simulink model "assignment_2_simulink_q710"  (R2023a)
settings: Solver=VariableStepAuto  StartTime=0.0  StopTime=0.5  MaxStep=1e-4  RelTol=1e-3
values from neighbouring files (symbols this model uses):
  J = 1e-3    (= 0.001)    [assignment_2_script_q6.m]    (also in assignment_2_script_q710.m)
  k = 0.35    [assignment_2_script_q6.m]    (also in assignment_2_script_q710.m)
  k_i = alpha_c^2 * L    (= 15791.3670417)    [assignment_2_script_q6.m]    (also in assignment_2_script_q710.m = 11053.9569292)
  k_is = alpha_s^2 * J    (= 63.165468167)    [assignment_2_script_q6.m]    (also in assignment_2_script_q710.m = 0)
  k_p = 2 * alpha_c* L - R    (= 12.0663706144)    [assignment_2_script_q6.m]    (also in assignment_2_script_q710.m = 8.04645943005)
  k_ps = 2 * alpha_s * J    (= 0.502654824574)    [assignment_2_script_q6.m]    (also in assignment_2_script_q710.m = 0.251327412287)
  k_t = alpha_c * L    (= 6.28318530718)    [assignment_2_script_q6.m]    (also in assignment_2_script_q710.m = 4.39822971503)
  k_ts = alpha_s * J    (= 0.251327412287)    [assignment_2_script_q6.m]    (also in assignment_2_script_q710.m)
  L = 2.5e-3    (= 0.0025)    [assignment_2_script_q6.m]    (also in assignment_2_script_q710.m = 0.00175)
  R = 0.5    [assignment_2_script_q6.m]    (also in assignment_2_script_q710.m = 0.75)
  tau_max = 2*tau_N    (= 14)    [assignment_2_script_q6.m]    (also in assignment_2_script_q710.m)
  tau_min = -2*tau_N    (= -14)    [assignment_2_script_q6.m]    (also in assignment_2_script_q710.m)
  u_max = 140    [assignment_2_script_q6.m]    (also in assignment_2_script_q710.m)
  u_min = -140    [assignment_2_script_q6.m]    (also in assignment_2_script_q710.m)
settings Model: Creator=chowd  LastModifiedBy=chowd
settings DataIOCC: ReturnWorkspaceOutputs=off

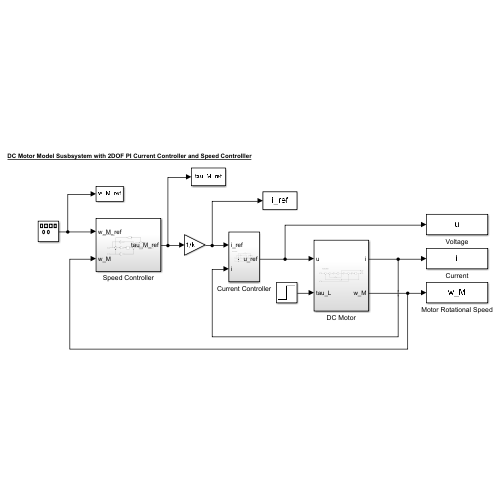
[thumbnail: Simulink's stored preview of the top-level diagram]
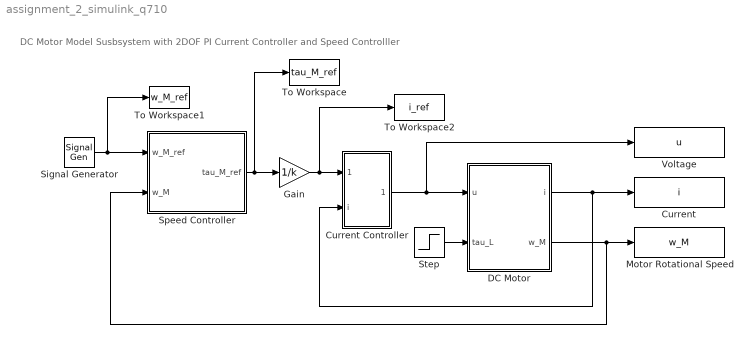
== system assignment_2_simulink_q710 ==
  note: DC Motor Model Susbsystem with 2DOF PI Current Controller and Speed Controlller
  Current : ToWorkspace  VariableName=i  SaveFormat=Timeseries  SampleTime=-1
  Current Controller : Subsystem
  DC Motor : Subsystem
  Gain : Gain  Gain=1/k
  Motor Rotational Speed : ToWorkspace  VariableName=w_M  SaveFormat=Timeseries  SampleTime=-1
  Signal Generator : SignalGenerator  WaveForm=square  Amplitude=160  Frequency=4
  Speed Controller : Subsystem
  Step : Step  Time=0.3  After=7  SampleTime=1
  To Workspace : ToWorkspace  VariableName=tau_M_ref  SaveFormat=Timeseries  SampleTime=-1
  To Workspace1 : ToWorkspace  VariableName=w_M_ref  SaveFormat=Timeseries  SampleTime=-1
  To Workspace2 : ToWorkspace  VariableName=i_ref  SaveFormat=Timeseries  SampleTime=-1
  Voltage : ToWorkspace  VariableName=u  SaveFormat=Timeseries  SampleTime=-1
  wires:
  Step/1 -> DC Motor/2(tau_L)
  Gain/1 -> To Workspace2/1, Current Controller/1(i_ref)
  DC Motor/1(i) -> Current/1, Current Controller/2(i)
  Current Controller/1(u_ref) -> Voltage/1, DC Motor/1(u)
  DC Motor/2(w_M) -> Speed Controller/2(w_M), Motor Rotational Speed/1
  Speed Controller/1(tau_M_ref) -> To Workspace/1, Gain/1
  Signal Generator/1 -> To Workspace1/1, Speed Controller/1(w_M_ref)

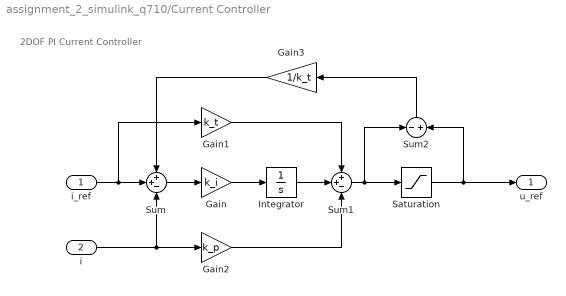
== system assignment_2_simulink_q710/Current Controller ==
  note: 2DOF PI Current Controller
  i_ref : Inport
  i : Inport  Port=2
  Gain : Gain  Gain=k_i
  Gain1 : Gain  Gain=k_t
  Gain2 : Gain  Gain=k_p
  Gain3 : Gain  Gain=1/k_t
  Integrator : Integrator
  Saturation : Saturate  UpperLimit=u_max  LowerLimit=u_min
  Sum : Sum  Inputs=++-
  Sum1 : Sum  Inputs=++-
  Sum2 : Sum  Inputs=-|+
  u_ref : Outport
  wires:
  i_ref/1 -> Sum/2, Gain1/1
  Saturation/1 -> u_ref/1, Sum2/2
  Gain3/1 -> Sum/1
  Integrator/1 -> Sum1/2
  Gain/1 -> Integrator/1
  Sum1/1 -> Sum2/1, Saturation/1
  Gain1/1 -> Sum1/1
  i/1 -> Sum/3, Gain2/1
  Sum/1 -> Gain/1
  Gain2/1 -> Sum1/3
  Sum2/1 -> Gain3/1

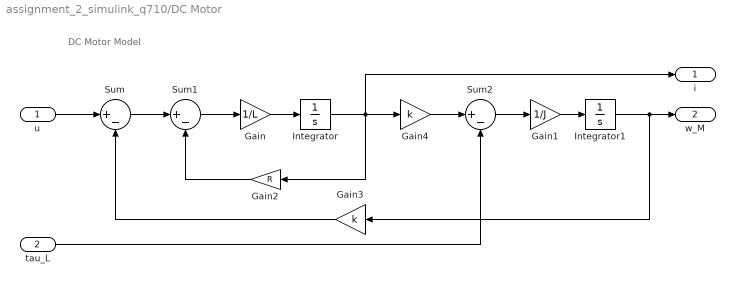
== system assignment_2_simulink_q710/DC Motor ==
  note: DC Motor Model
  u : Inport
  tau_L : Inport  Port=2
  Gain : Gain  Gain=1/L
  Gain1 : Gain  Gain=1/J
  Gain2 : Gain  Gain=R
  Gain3 : Gain  Gain=k
  Gain4 : Gain  Gain=k
  Integrator : Integrator
  Integrator1 : Integrator
  Sum : Sum  Inputs=|+-
  Sum1 : Sum  Inputs=|+-
  Sum2 : Sum  Inputs=|+-
  i : Outport
  w_M : Outport  Port=2
  wires:
  Gain/1 -> Integrator/1
  Sum2/1 -> Gain1/1
  Sum/1 -> Sum1/1
  u/1 -> Sum/1
  Integrator/1 -> Gain2/1, i/1, Gain4/1
  Sum1/1 -> Gain/1
  Gain2/1 -> Sum1/2
  Gain3/1 -> Sum/2
  tau_L/1 -> Sum2/2
  Integrator1/1 -> w_M/1, Gain3/1
  Gain4/1 -> Sum2/1
  Gain1/1 -> Integrator1/1

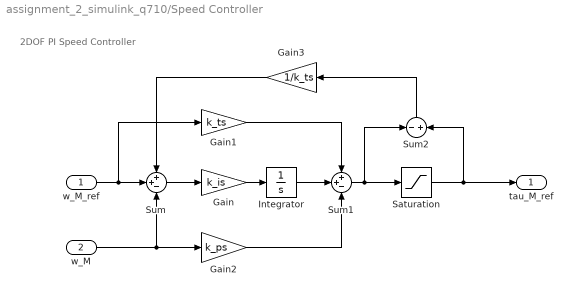
== system assignment_2_simulink_q710/Speed Controller ==
  note: 2DOF PI Speed Controller
  w_M_ref : Inport
  w_M : Inport  Port=2
  Gain : Gain  Gain=k_is
  Gain1 : Gain  Gain=k_ts
  Gain2 : Gain  Gain=k_ps
  Gain3 : Gain  Gain=1/k_ts
  Integrator : Integrator
  Saturation : Saturate  UpperLimit=tau_max  LowerLimit=tau_min
  Sum : Sum  Inputs=++-
  Sum1 : Sum  Inputs=++-
  Sum2 : Sum  Inputs=-|+
  tau_M_ref : Outport
  wires:
  w_M_ref/1 -> Sum/2, Gain1/1
  Saturation/1 -> tau_M_ref/1, Sum2/2
  Gain3/1 -> Sum/1
  Integrator/1 -> Sum1/2
  Gain/1 -> Integrator/1
  Sum1/1 -> Sum2/1, Saturation/1
  Gain1/1 -> Sum1/1
  w_M/1 -> Sum/3, Gain2/1
  Sum/1 -> Gain/1
  Gain2/1 -> Sum1/3
  Sum2/1 -> Gain3/1
